simulink model "KuehlungSpindel_P_Var"  (Simulink 7.6)
settings: Solver=ode45  StartTime=0.0  StopTime=SimulTime  RelTol=1e-3
values from neighbouring files (symbols this model uses):
  Ein = 1    [ParametersKuehlungSpindel_P_Var.m]
  EinAus = 1    [ParametersKuehlungSpindel_P_Var.m]
  f3 = 0.3252    [ParametersKuehlungSpindel_P_Var.m]
  geometrie = l    (= 0.314159265359)    [ParametersKuehlungSpindel_P_Var.m]
  MaxDrehmoment = 265    [ParametersKuehlungSpindel_P_Var.m]
  MaxDrehzahl = 6500    [ParametersKuehlungSpindel_P_Var.m]
  n = 0.8    [ParametersKuehlungSpindel_P_Var.m]
  n1 = 0.78    [ParametersKuehlungSpindel_P_Var.m]
  n2 = 0.7    [ParametersKuehlungSpindel_P_Var.m]
  p = 500    [ParametersKuehlungSpindel_P_Var.m]
  p1 = 380    [ParametersKuehlungSpindel_P_Var.m]
  p2 = 1100    [ParametersKuehlungSpindel_P_Var.m]
  PR = 1    [ParametersKuehlungSpindel_P_Var.m]
  Pr = 0.7    [ParametersKuehlungSpindel_P_Var.m]
  radius = 0.15    [ParametersKuehlungSpindel_P_Var.m]
  sb = 5.67*(10^-8)    (= 5.67e-08)    [ParametersKuehlungSpindel_P_Var.m]
  T_Umgebung = 296    [ParametersKuehlungSpindel_P_Var.m]
  Venti_n2 = 273+37    (= 310)    [ParametersKuehlungSpindel_P_Var.m]
undefined symbols (not defined in the file or in its folder): A, Job, KinematischeViskositaet, m, Schaltschrank_Kuehlung, Spindel, SpindelKuehlung, Temperatur, Waermeleitfaehigkeit
settings Model: Creator=conid  LastModifiedBy=conid

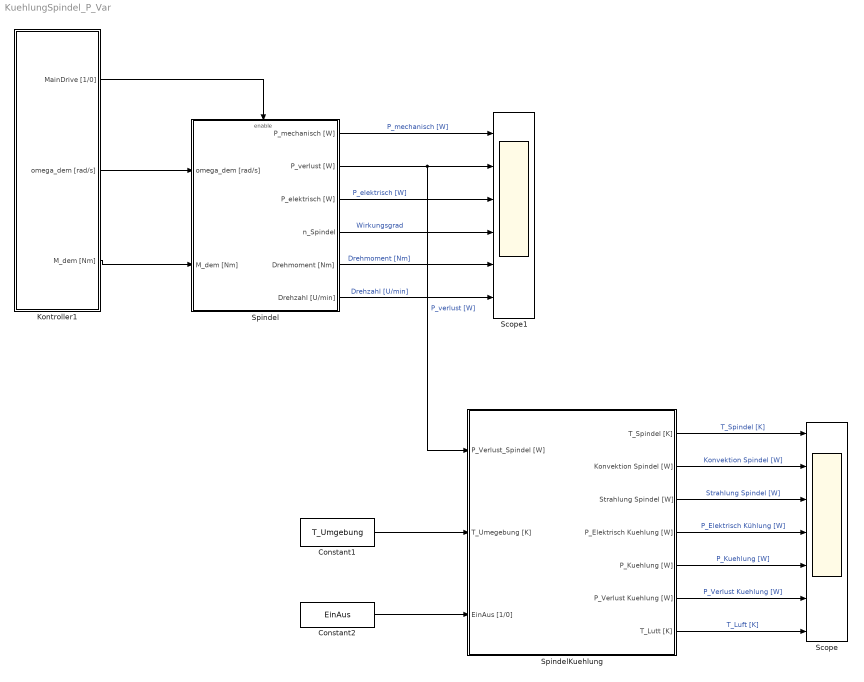
== system KuehlungSpindel_P_Var ==
  Constant1 : Constant  Value=T_Umgebung
  Constant2 : Constant  Value=EinAus
  Kontroller1 : Subsystem
  Scope : Scope  NumInputPorts=7
      settings: YMin=-5~-5~-5~-5~-5~-5~-5  YMax=5~5~5~5~5~5~5  SaveName=Scp_Cspindel
  Scope1 : Scope  NumInputPorts=6
      settings: TimeRange=100  YMin=0~-5000~-2000~-0.1~-5~-5  YMax=16000~30000~14000~0.9~5~5  SaveName=Scp_MainDrive
  Spindel : Subsystem  TreatAsAtomicUnit=on
  SpindelKuehlung : Subsystem  TreatAsAtomicUnit=on
  wires:
  SpindelKuehlung/1(T_Spindel [K]) -> Scope/1  "T_Spindel [K]"
  SpindelKuehlung/2(Konvektion Spindel [W]) -> Scope/2  "Konvektion Spindel [W]"
  SpindelKuehlung/3(Strahlung Spindel [W]) -> Scope/3  "Strahlung Spindel [W]"
  SpindelKuehlung/4(P_Elektrisch Kuehlung [W]) -> Scope/4  "P_Elektrisch Kühlung [W]"
  SpindelKuehlung/5(P_Kuehlung [W]) -> Scope/5  "P_Kuehlung [W]"
  SpindelKuehlung/6(P_Verlust Kuehlung [W]) -> Scope/6  "P_Verlust Kuehlung [W]"
  SpindelKuehlung/7(T_Lutt [K]) -> Scope/7  "T_Luft [K]"
  Spindel/1(P_mechanisch [W]) -> Scope1/1  "P_mechanisch [W]"
  Spindel/4(n_Spindel) -> Scope1/4  "Wirkungsgrad"
  Spindel/2(P_verlust [W]) -> Scope1/2, SpindelKuehlung/1(P_Verlust_Spindel [W])  "P_verlust [W]"
  Spindel/3(P_elektrisch [W]) -> Scope1/3  "P_elektrisch [W]"
  Kontroller1/2(omega_dem [rad/s]) -> Spindel/1(omega_dem [rad/s])
  Kontroller1/3(M_dem [Nm]) -> Spindel/2(M_dem [Nm])
  Kontroller1/1(MainDrive [1/0]) -> Spindel/Enable
  Spindel/5(Drehmoment [Nm]) -> Scope1/5  "Drehmoment [Nm]"
  Spindel/6(Drehzahl [U/min]) -> Scope1/6  "Drehzahl [U/min]"
  Constant1/1 -> SpindelKuehlung/2(T_Umegebung [K])
  Constant2/1 -> SpindelKuehlung/3(EinAus [1/0])

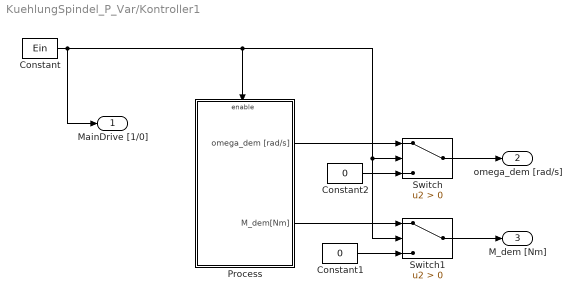
== system KuehlungSpindel_P_Var/Kontroller1 ==
  Constant : Constant  Value=Ein
  Constant1 : Constant  Value=0
  Constant2 : Constant  Value=0
  Process : Subsystem  TreatAsAtomicUnit=on
  Switch : Switch  Criteria=u2 > Threshold
  Switch1 : Switch  Criteria=u2 > Threshold
  MainDrive [1/0] : Outport
  omega_dem [rad/s] : Outport  Port=2
  M_dem [Nm] : Outport  Port=3
  wires:
  Constant/1 -> Process/Enable, Switch1/2, Switch/2, MainDrive [1/0]/1
  Process/1(omega_dem [rad/s]) -> Switch/1
  Process/2(M_dem[Nm]) -> Switch1/1
  Constant1/1 -> Switch1/3
  Switch/1 -> omega_dem [rad/s]/1
  Switch1/1 -> M_dem [Nm]/1
  Constant2/1 -> Switch/3

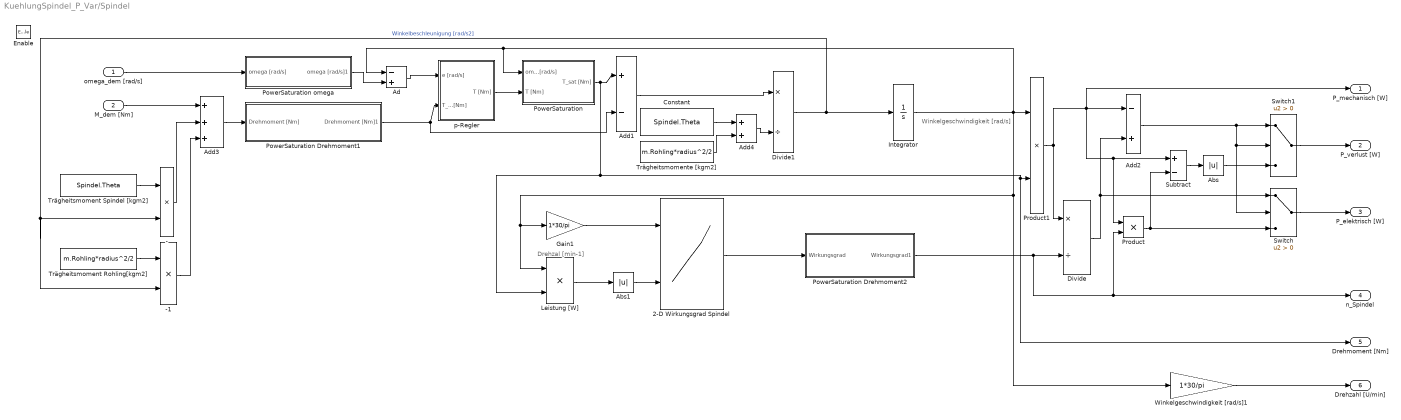
== system KuehlungSpindel_P_Var/Spindel ==
  note: Winkelgeschwindigkeit [rad/s]
  note: Drehzal [min-1]
  omega_dem [rad/s] : Inport
  M_dem [Nm] : Inport  Port=2
  Enable : EnablePort
  - : Product  RndMeth=Zero
  -1 : Product  RndMeth=Zero
  2-D Wirkungsgrad Spindel : Lookup_n-D  BreakpointsForDimension1=Spindel.Tabelleomega  BreakpointsForDimension2=Spindel.TabelleM  Table=Spindel.Tabelleeta  InterpMethod=Cubic spline  ExtrapMethod=None - Clip  RndMeth=Simplest  InputSameDT=on
  Abs : Abs
  Abs1 : Abs
  Ad : Sum  Inputs=-+
  Add1 : Sum  Inputs=+-
  Add2 : Sum  Inputs=-+
  Add3 : Sum  Inputs=+++
  Add4 : Sum
  Constant : Constant  Value=Spindel.Theta
  Divide : Product  Inputs=*/
  Divide1 : Product  Inputs=*/
  Gain1 : Gain  Gain=1*30/pi
  Integrator : Integrator
  Leistung [W] : Product  RndMeth=Zero
  PowerSaturation : Subsystem  TreatAsAtomicUnit=on
  PowerSaturation Drehmoment1 : Subsystem  TreatAsAtomicUnit=on
  PowerSaturation Drehmoment2 : Subsystem  TreatAsAtomicUnit=on
  PowerSaturation omega : Subsystem  TreatAsAtomicUnit=on
  Product : Product  RndMeth=Zero
  Product1 : Product  RndMeth=Zero
  Subtract : Sum  Inputs=+-
  Switch : Switch  Criteria=u2 > Threshold
  Switch1 : Switch  Criteria=u2 > Threshold
  Trägheitsmoment Rohling[kgm2] : Constant  Value=m.Rohling*radius^2/2
  Trägheitsmoment Spindel [kgm2] : Constant  Value=Spindel.Theta
  Trägheitsmomente [kgm2] : Constant  Value=m.Rohling*radius^2/2
  Winkelgeschwindigkeit [rad/s]1 : Gain  Gain=1*30/pi
  p-Regler : Subsystem  TreatAsAtomicUnit=on
  P_mechanisch [W] : Outport
  P_verlust [W] : Outport  Port=2
  P_elektrisch [W] : Outport  Port=3
  n_Spindel : Outport  Port=4
  Drehmoment [Nm] : Outport  Port=5
  Drehzahl [U/min] : Outport  Port=6
  wires:
  Ad/1 -> p-Regler/1(e [rad/s])
  p-Regler/1(T [Nm]) -> PowerSaturation/2(T [Nm])
  PowerSaturation/1(T_sat [Nm]) -> Leistung [W]/2, Product1/2, Drehmoment [Nm]/1, Add1/1
  Integrator/1 -> Product1/1, Ad/1, PowerSaturation/1(omega [rad/s]), Leistung [W]/1, Gain1/1, Winkelgeschwindigkeit [rad/s]1/1
  Product1/1 -> Divide/1, Add2/1, P_mechanisch [W]/1, Subtract/1, Product/1
  Divide/1 -> Add2/2, Switch/1
  Gain1/1 -> 2-D Wirkungsgrad Spindel/1
  Trägheitsmoment Spindel [kgm2]/1 -> -/1
  M_dem [Nm]/1 -> Add3/1
  -/1 -> Add3/2
  -1/1 -> Add3/3
  Trägheitsmoment Rohling[kgm2]/1 -> -1/1
  Add1/1 -> Divide1/1
  Divide1/1 -> Integrator/1, -1/2, -/2  "Winkelbeschleunigung [rad/s2]"
  Add4/1 -> Divide1/2
  Constant/1 -> Add4/1
  Trägheitsmomente [kgm2]/1 -> Add4/2
  Switch1/1 -> P_verlust [W]/1
  Switch/1 -> P_elektrisch [W]/1
  Add2/1 -> Switch1/1, Switch1/2, Switch/2
  Product/1 -> Subtract/2, Switch/3
  Subtract/1 -> Abs/1
  Abs/1 -> Switch1/3
  Abs1/1 -> 2-D Wirkungsgrad Spindel/2
  Leistung [W]/1 -> Abs1/1
  Winkelgeschwindigkeit [rad/s]1/1 -> Drehzahl [U/min]/1
  Add3/1 -> PowerSaturation Drehmoment1/1(Drehmoment [Nm])
  PowerSaturation Drehmoment1/1(Drehmoment [Nm]1) -> Add1/2, p-Regler/2(T_dem [Nm])
  omega_dem [rad/s]/1 -> PowerSaturation omega/1(omega [rad/s])
  PowerSaturation omega/1(omega [rad/s]1) -> Ad/2
  2-D Wirkungsgrad Spindel/1 -> PowerSaturation Drehmoment2/1(Wirkungsgrad)
  PowerSaturation Drehmoment2/1(Wirkungsgrad1) -> Divide/2, Product/2, n_Spindel/1

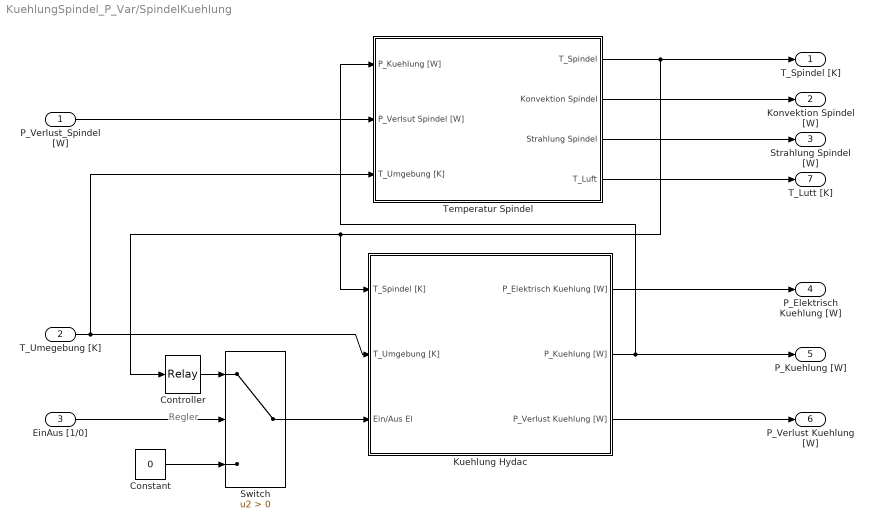
== system KuehlungSpindel_P_Var/SpindelKuehlung ==
  note: Regler
  P_Verlust_Spindel [W] : Inport
  T_Umegebung [K] : Inport  Port=2
  EinAus [1/0] : Inport  Port=3
  Constant : Constant  Value=0
  Controller : Relay  OnSwitchValue=Schaltschrank_Kuehlung.Tmax  OffSwitchValue=Schaltschrank_Kuehlung.Tmin
  Kuehlung Hydac : Subsystem
  Switch : Switch  Criteria=u2 > Threshold
  Temperatur Spindel : Subsystem
  T_Spindel [K] : Outport
  Konvektion Spindel [W] : Outport  Port=2
  Strahlung Spindel [W] : Outport  Port=3
  P_Elektrisch Kuehlung [W] : Outport  Port=4
  P_Kuehlung [W] : Outport  Port=5
  P_Verlust Kuehlung [W] : Outport  Port=6
  T_Lutt [K] : Outport  Port=7
  wires:
  Controller/1 -> Switch/1
  Temperatur Spindel/1(T_Spindel) -> Controller/1, Kuehlung Hydac/1(T_Spindel [K]), T_Spindel [K]/1
  T_Umegebung [K]/1 -> Kuehlung Hydac/2(T_Umgebung [K]), Temperatur Spindel/3(T_Umgebung [K])
  Kuehlung Hydac/2(P_Kuehlung [W]) -> Temperatur Spindel/1(P_Kuehlung [W]), P_Kuehlung [W]/1
  Temperatur Spindel/2(Konvektion Spindel) -> Konvektion Spindel [W]/1
  Temperatur Spindel/3(Strahlung Spindel) -> Strahlung Spindel [W]/1
  Kuehlung Hydac/1(P_Elektrisch Kuehlung [W]) -> P_Elektrisch Kuehlung [W]/1
  Kuehlung Hydac/3(P_Verlust Kuehlung [W]) -> P_Verlust Kuehlung [W]/1
  P_Verlust_Spindel [W]/1 -> Temperatur Spindel/2(P_Verlsut Spindel [W])
  Temperatur Spindel/4(T_Luft) -> T_Lutt [K]/1
  Constant/1 -> Switch/3
  EinAus [1/0]/1 -> Switch/2
  Switch/1 -> Kuehlung Hydac/3(Ein/Aus El)

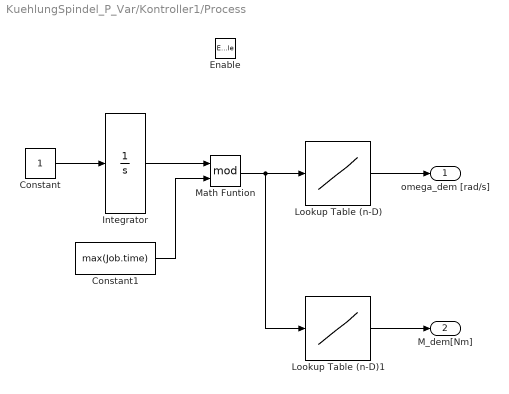
== system KuehlungSpindel_P_Var/Kontroller1/Process ==
  Enable : EnablePort
  Constant : Constant
  Constant1 : Constant  Value=max(Job.time)
  Integrator : Integrator
  Lookup Table (n-D) : Lookup_n-D  NumberOfTableDimensions=1  BreakpointsForDimension1=Job.time  Table=Job.omega_dem  InterpMethod=None - Flat  ExtrapMethod=Cubic spline  InputSameDT=on
  Lookup Table (n-D)1 : Lookup_n-D  NumberOfTableDimensions=1  BreakpointsForDimension1=Job.time  Table=Job.M_dem  InterpMethod=None - Flat  InputSameDT=on
  Math Funtion : Math  Operator=mod  SaturateOnIntegerOverflow=on
  omega_dem [rad/s] : Outport
  M_dem[Nm] : Outport  Port=2
  wires:
  Constant/1 -> Integrator/1
  Integrator/1 -> Math Funtion/1
  Math Funtion/1 -> Lookup Table (n-D)/1, Lookup Table (n-D)1/1
  Lookup Table (n-D)/1 -> omega_dem [rad/s]/1
  Lookup Table (n-D)1/1 -> M_dem[Nm]/1
  Constant1/1 -> Math Funtion/2

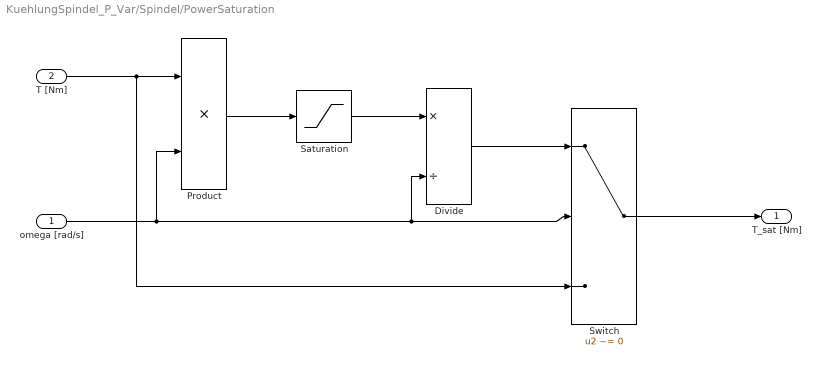
== system KuehlungSpindel_P_Var/Spindel/PowerSaturation ==
  omega [rad/s] : Inport
  T [Nm] : Inport  Port=2
  Divide : Product  Inputs=*/
  Product : Product  RndMeth=Zero
  Saturation : Saturate  UpperLimit=Spindel.Pmax  LowerLimit=-Spindel.Pmax
  Switch : Switch  Criteria=u2 ~= 0
  T_sat [Nm] : Outport
  wires:
  Product/1 -> Saturation/1
  Saturation/1 -> Divide/1
  Divide/1 -> Switch/1
  Switch/1 -> T_sat [Nm]/1
  T [Nm]/1 -> Product/1, Switch/3
  omega [rad/s]/1 -> Switch/2, Divide/2, Product/2

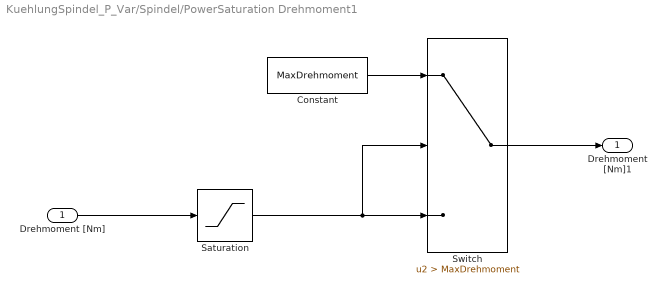
== system KuehlungSpindel_P_Var/Spindel/PowerSaturation Drehmoment1 ==
  Drehmoment [Nm] : Inport
  Constant : Constant  Value=MaxDrehmoment
  Saturation : Saturate  UpperLimit=MaxDrehmoment  LowerLimit=-MaxDrehmoment  ZeroCross=off
  Switch : Switch  Criteria=u2 > Threshold  Threshold=MaxDrehmoment
  Drehmoment [Nm]1 : Outport
  wires:
  Saturation/1 -> Switch/3, Switch/2
  Constant/1 -> Switch/1
  Drehmoment [Nm]/1 -> Saturation/1
  Switch/1 -> Drehmoment [Nm]1/1

== system KuehlungSpindel_P_Var/Spindel/PowerSaturation Drehmoment2 ==
  Wirkungsgrad : Inport
  Saturation : Saturate  UpperLimit=0.95  LowerLimit=0.1  ZeroCross=off
  Wirkungsgrad1 : Outport
  wires:
  Wirkungsgrad/1 -> Saturation/1
  Saturation/1 -> Wirkungsgrad1/1

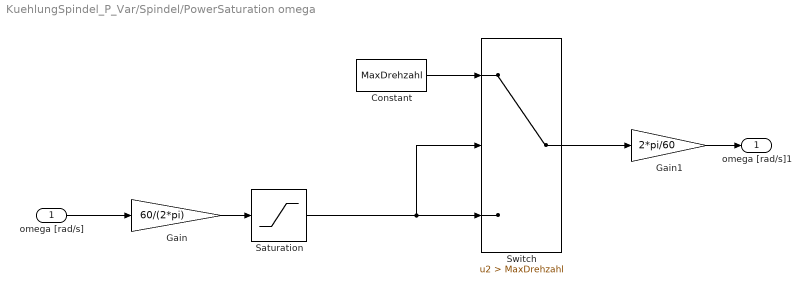
== system KuehlungSpindel_P_Var/Spindel/PowerSaturation omega ==
  omega [rad/s] : Inport
  Constant : Constant  Value=MaxDrehzahl
  Gain : Gain  Gain=60/(2*pi)
  Gain1 : Gain  Gain=2*pi/60
  Saturation : Saturate  UpperLimit=MaxDrehzahl  LowerLimit=0  ZeroCross=off
  Switch : Switch  Criteria=u2 > Threshold  Threshold=MaxDrehzahl
  omega [rad/s]1 : Outport
  wires:
  Saturation/1 -> Switch/3, Switch/2
  Constant/1 -> Switch/1
  omega [rad/s]/1 -> Gain/1
  Switch/1 -> Gain1/1
  Gain1/1 -> omega [rad/s]1/1
  Gain/1 -> Saturation/1

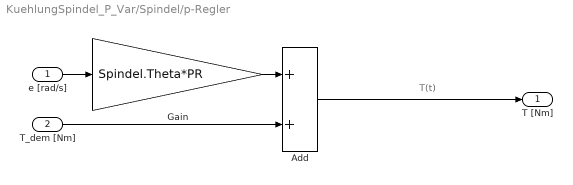
== system KuehlungSpindel_P_Var/Spindel/p-Regler ==
  note: T(t)
  e [rad/s] : Inport
  T_dem [Nm] : Inport  Port=2
  Add : Sum
  Gain : Gain  Gain=Spindel.Theta*PR
  T [Nm] : Outport
  wires:
  Add/1 -> T [Nm]/1
  T_dem [Nm]/1 -> Add/2
  Gain/1 -> Add/1
  e [rad/s]/1 -> Gain/1

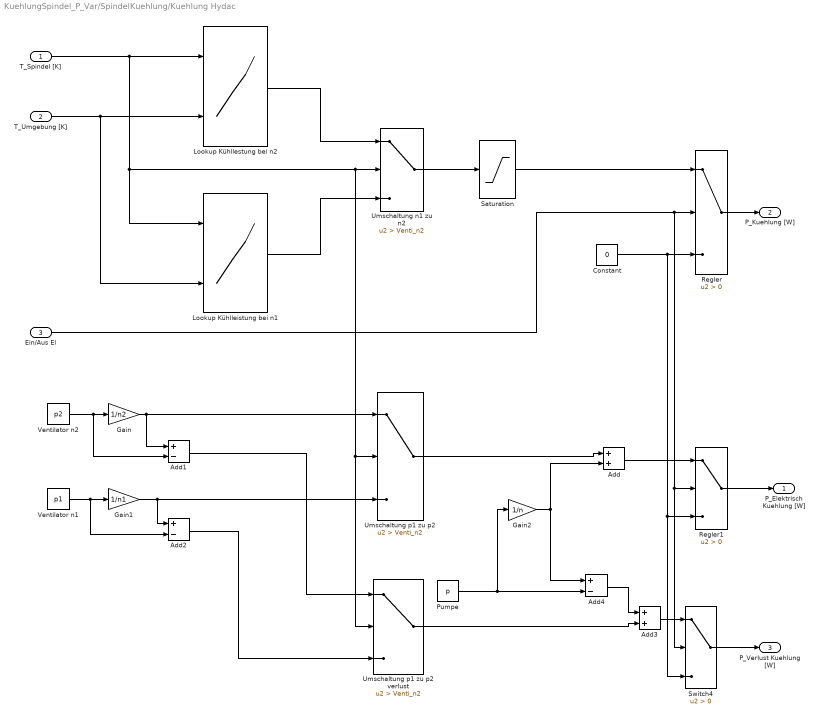
== system KuehlungSpindel_P_Var/SpindelKuehlung/Kuehlung Hydac ==
  T_Spindel [K] : Inport
  T_Umgebung [K] : Inport  Port=2
  Ein/Aus El : Inport  Port=3
  Add : Sum
  Add1 : Sum  Inputs=+-
  Add2 : Sum  Inputs=+-
  Add3 : Sum
  Add4 : Sum  Inputs=+-
  Constant : Constant  Value=0
  Gain : Gain  Gain=1/n2
  Gain1 : Gain  Gain=1/n1
  Gain2 : Gain  Gain=1/n
  Lookup Kühlleistung bei n1 : Lookup_n-D  BreakpointsForDimension1=SpindelKuehlung.Fluid.T_int  BreakpointsForDimension2=SpindelKuehlung.Luft.T_ext  Table=SpindelKuehlung.P  InterpMethod=Cubic spline  ExtrapMethod=None - Clip  InputSameDT=on
  Lookup Kühllestung bei n2 : Lookup_n-D  BreakpointsForDimension1=SpindelKuehlung.Fluid.T_int  BreakpointsForDimension2=SpindelKuehlung.Luft.T_ext  Table=SpindelKuehlung.P_n2  InterpMethod=Cubic spline  ExtrapMethod=None - Clip  InputSameDT=on
  Pumpe : Constant  Value=p
  Regler : Switch  Criteria=u2 > Threshold
  Regler1 : Switch  Criteria=u2 > Threshold
  Saturation : Saturate  UpperLimit=12000  LowerLimit=0
  Switch4 : Switch  Criteria=u2 > Threshold
  Umschaltung n1 zu n2 : Switch  Criteria=u2 > Threshold  Threshold=Venti_n2
  Umschaltung p1 zu p2 : Switch  Criteria=u2 > Threshold  Threshold=Venti_n2
  Umschaltung p1 zu p2 verlust : Switch  Criteria=u2 > Threshold  Threshold=Venti_n2
  Ventilator n1 : Constant  Value=p1
  Ventilator n2 : Constant  Value=p2
  P_Elektrisch Kuehlung [W] : Outport
  P_Kuehlung [W] : Outport  Port=2
  P_Verlust Kuehlung [W] : Outport  Port=3
  wires:
  Constant/1 -> Regler/3, Regler1/3, Switch4/3
  Saturation/1 -> Regler/1
  Regler/1 -> P_Kuehlung [W]/1
  T_Spindel [K]/1 -> Lookup Kühllestung bei n2/1, Lookup Kühlleistung bei n1/1, Umschaltung n1 zu n2/2, Umschaltung p1 zu p2/2, Umschaltung p1 zu p2 verlust/2
  Ein/Aus El/1 -> Regler/2, Regler1/2, Switch4/2
  T_Umgebung [K]/1 -> Lookup Kühllestung bei n2/2, Lookup Kühlleistung bei n1/2
  Lookup Kühllestung bei n2/1 -> Umschaltung n1 zu n2/1
  Lookup Kühlleistung bei n1/1 -> Umschaltung n1 zu n2/3
  Umschaltung p1 zu p2/1 -> Add/1
  Ventilator n2/1 -> Gain/1, Add1/2
  Gain/1 -> Umschaltung p1 zu p2/1, Add1/1
  Gain1/1 -> Umschaltung p1 zu p2/3, Add2/1
  Ventilator n1/1 -> Gain1/1, Add2/2
  Gain2/1 -> Add/2, Add4/1
  Pumpe/1 -> Gain2/1, Add4/2
  Add4/1 -> Add3/1
  Add1/1 -> Umschaltung p1 zu p2 verlust/1
  Add2/1 -> Umschaltung p1 zu p2 verlust/3
  Umschaltung p1 zu p2 verlust/1 -> Add3/2
  Add/1 -> Regler1/1
  Regler1/1 -> P_Elektrisch Kuehlung [W]/1
  Add3/1 -> Switch4/1
  Switch4/1 -> P_Verlust Kuehlung [W]/1
  Umschaltung n1 zu n2/1 -> Saturation/1

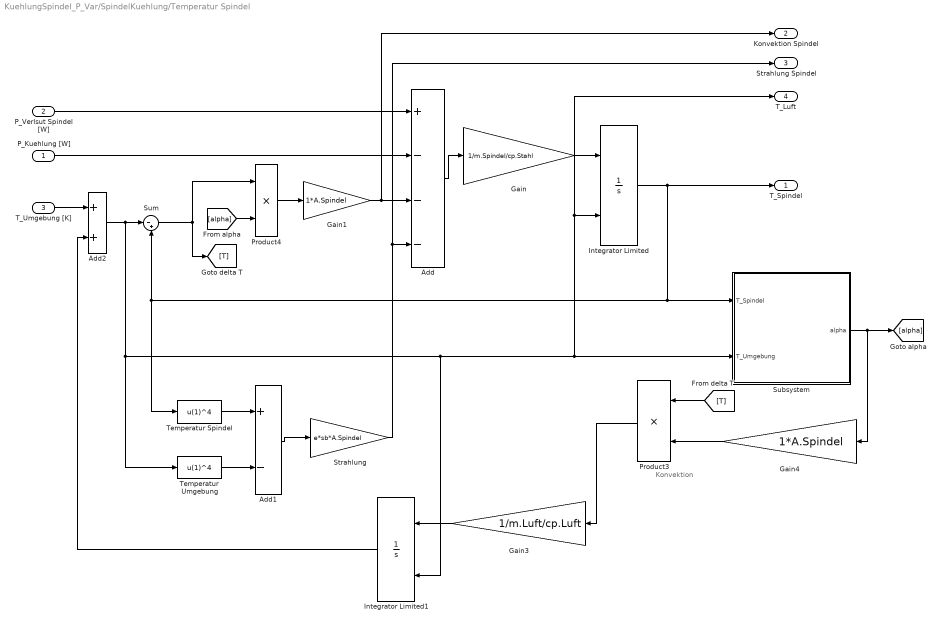
== system KuehlungSpindel_P_Var/SpindelKuehlung/Temperatur Spindel ==
  note: Konvektion
  P_Kuehlung [W] : Inport
  P_Verlsut Spindel [W] : Inport  Port=2
  T_Umgebung [K] : Inport  Port=3
  Add : Sum  Inputs=+---
  Add1 : Sum  Inputs=+-
  Add2 : Sum
  Gain : Gain  Gain=1/m.Spindel/cp.Stahl
  Gain1 : Gain  Gain=1*A.Spindel
  Gain3 : Gain  Gain=1/m.Luft/cp.Luft
  Gain4 : Gain  Gain=1*A.Spindel
  Integrator Limited : Integrator  InitialConditionSource=external  LimitOutput=on  ZeroCross=off
  Integrator Limited1 : Integrator  InitialConditionSource=external  LimitOutput=on  ZeroCross=off
  Product3 : Product  RndMeth=Zero
  Product4 : Product  RndMeth=Zero
  Strahlung : Gain  Gain=e*sb*A.Spindel
  Subsystem : Subsystem
  Sum : Sum  Inputs=|-+
  Temperatur Spindel : Fcn  Expr=u(1)^4
  Temperatur Umgebung : Fcn  Expr=u(1)^4
  T_Spindel : Outport
  Konvektion Spindel : Outport  Port=2
  Strahlung Spindel : Outport  Port=3
  T_Luft : Outport  Port=4
  wires:
  P_Verlsut Spindel [W]/1 -> Add/1
  Sum/1 -> Product4/1, [T]
  Gain/1 -> Integrator Limited/1
  Gain1/1 -> Konvektion Spindel/1, Add/3
  Integrator Limited/1 -> T_Spindel/1, Sum/2, Temperatur Spindel/1, Subsystem/1(T_Spindel)
  Add/1 -> Gain/1
  Strahlung/1 -> Strahlung Spindel/1, Add/4
  Temperatur Spindel/1 -> Add1/1
  Temperatur Umgebung/1 -> Add1/2
  Add1/1 -> Strahlung/1
  Add2/1 -> Sum/1, Temperatur Umgebung/1, Integrator Limited/2, T_Luft/1, Subsystem/2(T_Umgebung), Integrator Limited1/2
  T_Umgebung [K]/1 -> Add2/1
  Subsystem/1(alpha) -> Gain4/1, [alpha]
  Product4/1 -> Gain1/1
  [alpha] -> Product4/2
  Gain4/1 -> Product3/2
  [T] -> Product3/1
  P_Kuehlung [W]/1 -> Add/2
  Gain3/1 -> Integrator Limited1/1
  Integrator Limited1/1 -> Add2/2
  Product3/1 -> Gain3/1

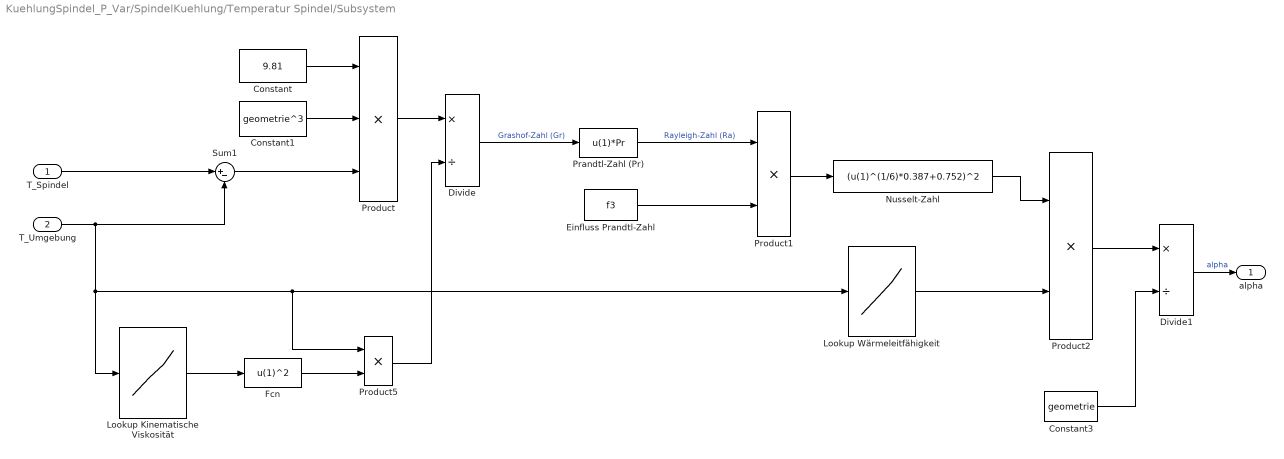
== system KuehlungSpindel_P_Var/SpindelKuehlung/Temperatur Spindel/Subsystem ==
  T_Spindel : Inport
  T_Umgebung : Inport  Port=2
  Constant : Constant  Value=9.81
  Constant1 : Constant  Value=geometrie^3
  Constant3 : Constant  Value=geometrie
  Divide : Product  Inputs=*/
  Divide1 : Product  Inputs=*/
  Einfluss Prandtl-Zahl : Constant  Value=f3
  Fcn : Fcn  Expr=u(1)^2
  Lookup Kinematische Viskosität : Lookup_n-D  NumberOfTableDimensions=1  BreakpointsForDimension1=Temperatur.Tabel  Table=KinematischeViskositaet.Tabel  InterpMethod=Cubic spline  ExtrapMethod=None - Clip  InputSameDT=on
  Lookup Wärmeleitfähigkeit : Lookup_n-D  NumberOfTableDimensions=1  BreakpointsForDimension1=Temperatur.Tabel  Table=Waermeleitfaehigkeit.Tabel  InterpMethod=Cubic spline  ExtrapMethod=None - Clip  InputSameDT=on
  Nusselt-Zahl : Fcn  Expr=(u(1)^(1/6)*0.387+0.752)^2
  Prandtl-Zahl (Pr) : Fcn  Expr=u(1)*Pr
  Product : Product  Inputs=3  RndMeth=Zero
  Product1 : Product  RndMeth=Zero
  Product2 : Product  RndMeth=Zero
  Product5 : Product  RndMeth=Zero
  Sum1 : Sum  Inputs=|+-
  alpha : Outport
  wires:
  Constant/1 -> Product/1
  Constant1/1 -> Product/2
  Sum1/1 -> Product/3
  Product/1 -> Divide/1
  Divide/1 -> Prandtl-Zahl (Pr)/1  "Grashof-Zahl (Gr)"
  Prandtl-Zahl (Pr)/1 -> Product1/1  "Rayleigh-Zahl (Ra)"
  Einfluss Prandtl-Zahl/1 -> Product1/2
  Lookup Wärmeleitfähigkeit/1 -> Product2/2
  Product2/1 -> Divide1/1
  Product5/1 -> Divide/2
  Lookup Kinematische Viskosität/1 -> Fcn/1
  Fcn/1 -> Product5/2
  Product1/1 -> Nusselt-Zahl/1
  Nusselt-Zahl/1 -> Product2/1
  Constant3/1 -> Divide1/2
  T_Spindel/1 -> Sum1/1
  T_Umgebung/1 -> Sum1/2, Lookup Kinematische Viskosität/1, Product5/1, Lookup Wärmeleitfähigkeit/1
  Divide1/1 -> alpha/1  "alpha"
